simulink model "HumanPilot"  (R2023b)
settings: Solver=FixedStepAuto  StartTime=0.0  StopTime=inf  FixedStep=sample_time  RelTol=1e-3
model workspace (MAT data in the model file):
  SL_ROS_VariableLengthArrays_MaxSizes.CommonInfo.ArrayTruncateAction = 'EmitWarning'
  SL_ROS_VariableLengthArrays_MaxSizes.MsgTypeMap = containers.Map
  SL_ROS_VariableLengthArrays_MaxSizes.MsgTypeMap.serialization.keys = {'sensor_msgs/Image'}
  SL_ROS_VariableLengthArrays_MaxSizes.MsgTypeMap.serialization.values{1}(1).PropertyName = 'data'
  SL_ROS_VariableLengthArrays_MaxSizes.MsgTypeMap.serialization.values{1}(1).DataType = 'uint8'
  SL_ROS_VariableLengthArrays_MaxSizes.MsgTypeMap.serialization.values{1}(1).MaxLength = 921600
  SL_ROS_VariableLengthArrays_MaxSizes.MsgTypeMap.serialization.values{1}(2).PropertyName = 'encoding'
  SL_ROS_VariableLengthArrays_MaxSizes.MsgTypeMap.serialization.values{1}(2).DataType = 'uint8'
  SL_ROS_VariableLengthArrays_MaxSizes.MsgTypeMap.serialization.values{1}(2).MaxLength = 128
  SL_ROS_VariableLengthArrays_MaxSizes.MsgTypeMap.serialization.uniformity = 0
  SL_ROS_VariableLengthArrays_MaxSizes.MsgTypeMap.serialization.keyType = 'char'
  SL_ROS_VariableLengthArrays_MaxSizes.MsgTypeMap.serialization.valueType = 'any'
  sample_time = 0.1
undefined symbols (not defined in the file): duration, vel
libraries: ros2lib x6, visionsinks x2, vrlib x1, simulink_extras x1
settings Model: Creator=rcasado  LastModifiedBy=Rafa
settings SolverCC: AlgebraicLoopSolver=TrustRegion
settings DataIOCC: ReturnWorkspaceOutputs=off
settings OptimizationCC: EnhancedBackFolding=on  PassReuseOutputArgsAs=Individual arguments  ZeroExternalMemoryAtStartup=off  ZeroInternalMemoryAtStartup=off  MaxStackSize=64  OptimizeBlockOrder=speed  DifferentSizesBufferReuse=on  OptimizationCustomize=off  EfficientTunableParamExpr=on
settings DebuggingCC: ParameterTunabilityLossMsg=error  UnconnectedInputMsg=warning  UnconnectedOutputMsg=warning  UnconnectedLineMsg=warning  BusObjectLabelMismatch=none  PregeneratedLibrarySubsystemCodeDiagnostic=none  ArithmeticOperatorsInVariantConditions=warning
settings HardwareCC: ProdBitPerPointer=32  ProdBitPerSizeT=32  ProdBitPerPtrDiffT=32  ProdLargestAtomicFloat=None  ProdIntDivRoundTo=Undefined  ProdEndianess=Unspecified  ProdWordSize=32  ProdHWDeviceType=Generic->Unspecified (assume 32-bit Generic)
settings ModelReferenceCC: EnableRefExpFcnMdlSchedulingChecks=on
settings SFSimCC: SimUseLocalCustomCode=off  CustomCodeUndefinedFunction=UseInterfaceOnly  SimTargetLang=C++
settings RTWCC: Description=Embedded Coder  SystemTargetFile=ert.tlc  HardwareBoard=Robot Operating System (ROS)  TLCOptions="-aInlineSetEventsForThisBaseRateFcn=TLC_FALSE -aSuppressMultiTaskScheduler=TLC_FALSE  -aRateBasedStepFcn=0"  TemplateMakefile=ert_default_tmf  GenerateReport=on  RTWUseLocalCustomCode=off  Toolchain=Catkin  IncludeHyperlinkInReport=on  LaunchReport=on  TargetLang=C++  GenerateTraceInfo=on  GenerateTraceReport=on  GenerateTraceReportSl=on  GenerateTraceReportSf=on  GenerateTraceReportEml=on  DLArmComputeVersion=19.05
settings CodeAppCC: ForceParamTrailComments=on  IgnoreCustomStorageClasses=off  OperatorAnnotations=on  SimulinkDataObjDesc=on  SFDataObjDesc=on  InsertBlockDesc=on

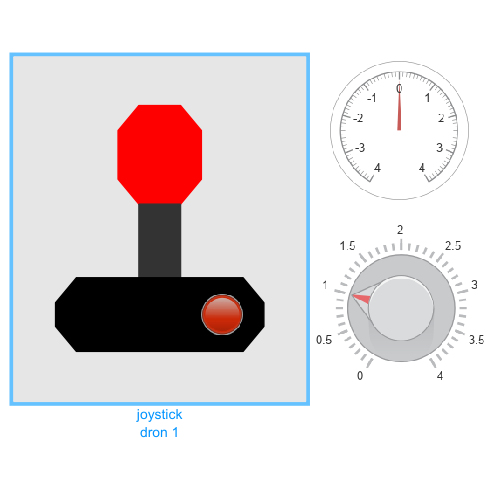
[thumbnail: Simulink's stored preview of the top-level diagram]
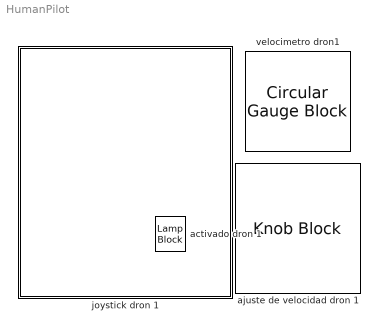
== system HumanPilot ==
  activado dron 1 : LampBlock  LabelPosition=Hide
  ajuste de velocidad dron 1 : KnobBlock  LabelPosition=Hide  ScaleMax=4  TickInterval=0.5
  joystick dron 1 : Subsystem
      mask Display:
      | patch([12 -2 -2 12], [12 12 -2 -2], [0.9 0.9 0.9])
      | 
      | % bola roja
      | patch([4 6 7 7 6 4 3 3], [6 6 7 9 10 10 9 7], [1 0 0])
      | 
      | % palo gris
      | patch([4 6 6 4], [3 3 6 6], [0.2 0.2 0.2])
      | 
      | % base negra
      | patch([1 9 10 10 9 1 0 0], [0 0 1 2 3 3 2 1], [0 0 0])
  velocimetro dron1 : CircularGaugeBlock  LabelPosition=Hide  ScaleMin=-4  ScaleMax=4  TickInterval=1

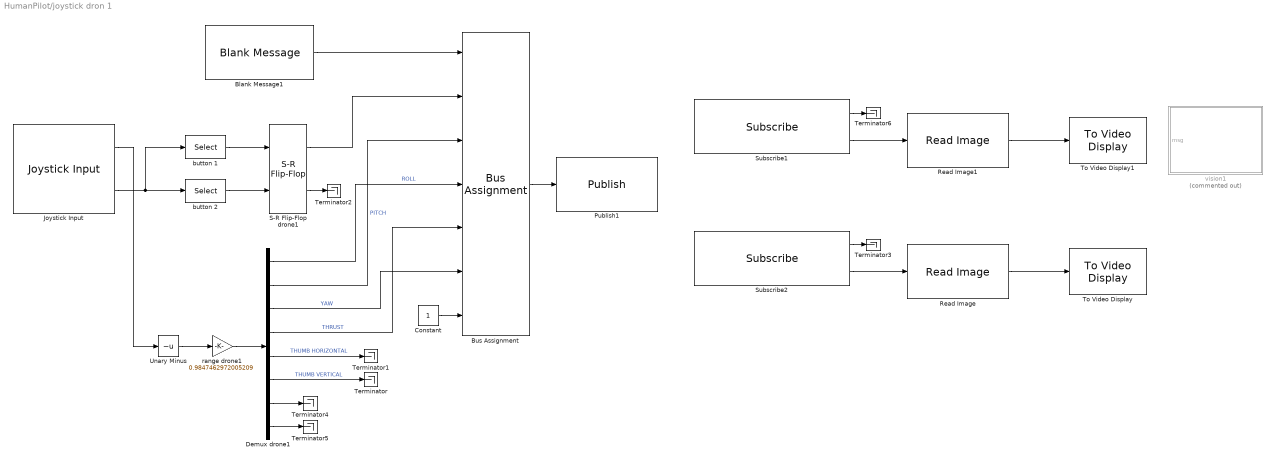
== system HumanPilot/joystick dron 1 ==
  Blank Message1 : ros2lib/Blank Message  messageClass=Message  entityType=navsim_msgs/RemoteCommand  messageType=navsim_msgs/RemoteCommand  SampleTime=sample_time
  Bus Assignment : BusAssignment  AssignedSignals=on,vel.linear.x,vel.linear.y,vel.linear.z,vel.angular.z,duration.sec
  Constant : Constant  OutDataTypeStr=int32
  Demux drone1 : Demux  Outputs=8
  Joystick Input : vrlib/Joystick Input  joyid=1  adjustports=off  forcefeed=off
  Publish1 : ros2lib/Publish  topicSource=Select from ROS network  topic=/UAV/abejorro1/RemoteCommand  messageType=navsim_msgs/RemoteCommand  QOSHistory=Keep last  QOSDepth=1  QOSReliability=Reliable  QOSDurability=Volatile
  Read Image : ros2lib/Read Image  MaximumImageSize=[320, 480]  ImageEncoding=rgb8  ShowAlphaOutput=off  ShowErrorCodeOutput=off  VariableSizeOutputs=off
  Read Image1 : ros2lib/Read Image  MaximumImageSize=[240, 320]  ImageEncoding=rgb8  ShowAlphaOutput=off  ShowErrorCodeOutput=off  VariableSizeOutputs=off
  S-R Flip-Flop drone1 : simulink_extras/Flip Flops/S-R Flip-Flop  initial_condition=0
  Subscribe1 : ros2lib/Subscribe  topicSource=Select from ROS network  topic=/UAV/abejorro1/onboard_cam/image_raw  messageType=sensor_msgs/Image  sampleTime=0.1  QOSHistory=Keep last  QOSDepth=1  QOSReliability=Reliable  QOSDurability=Volatile
  Subscribe2 : ros2lib/Subscribe  topicSource=Select from ROS network  topic=/UAV/abejorro1/follow_cam/image_raw  messageType=sensor_msgs/Image  sampleTime=0.1  QOSHistory=Keep last  QOSDepth=1  QOSReliability=Reliable  QOSDurability=Volatile
  Terminator{,1..6} (7 alike) : Terminator
  To Video Display : visionsinks/To Video Display  windowSizeMode=True size (1:1)  openAtMdlStart=on  fullScreen=off  videoWindowX=4122  videoWindowY=1148  saveWindowSize=off  videoWindowWidth=480  videoWindowHeight=320  inputColorFormat=RGB  inputType=Obsolete  imagePorts=One multidimensional signal  OutputDevice=On-screen video monitor  dataOrg=Column-major  isWindowOpen=off
  To Video Display1 : visionsinks/To Video Display  windowSizeMode=Normal  openAtMdlStart=on  fullScreen=off  videoWindowX=3600  videoWindowY=1154  saveWindowSize=off  videoWindowWidth=430  videoWindowHeight=322  inputColorFormat=RGB  inputType=Obsolete  imagePorts=One multidimensional signal  OutputDevice=On-screen video monitor  dataOrg=Column-major  isWindowOpen=off
  Unary Minus : UnaryMinus
  button 1 : Selector  InputPortWidth=32  IndexOptions=Index vector (dialog)  Indices=[1]  OutputSizes=1
  button 2 : Selector  InputPortWidth=32  IndexOptions=Index vector (dialog)  Indices=[2]  OutputSizes=1
  range drone1 : Gain  Gain=0.9847462972005209
  vision1 : MATLAB Function  Commented=on  TreatAsAtomicUnit=on
  wires:
  Bus Assignment/1 -> Publish1/1
  Blank Message1/1 -> Bus Assignment/1
  Joystick Input/1 -> Unary Minus/1
  Demux drone1/1 -> Bus Assignment/4  "ROLL"
  Demux drone1/2 -> Bus Assignment/3  "PITCH"
  Demux drone1/3 -> Bus Assignment/6  "YAW"
  Demux drone1/4 -> Bus Assignment/5  "THRUST"
  Demux drone1/5 -> Terminator1/1  "THUMB HORIZONTAL"
  Demux drone1/6 -> Terminator/1  "THUMB VERTICAL"
  Demux drone1/7 -> Terminator4/1
  Demux drone1/8 -> Terminator5/1
  Joystick Input/2 -> button 2/1, button 1/1
  S-R Flip-Flop drone1/1 -> Bus Assignment/2
  button 2/1 -> S-R Flip-Flop drone1/2
  button 1/1 -> S-R Flip-Flop drone1/1
  S-R Flip-Flop drone1/2 -> Terminator2/1
  Unary Minus/1 -> range drone1/1
  range drone1/1 -> Demux drone1/1
  Subscribe1/2 -> Read Image1/1
  Read Image1/1 -> To Video Display1/1
  Subscribe1/1 -> Terminator6/1
  Subscribe2/1 -> Terminator3/1
  Subscribe2/2 -> Read Image/1
  Read Image/1 -> To Video Display/1
  Constant/1 -> Bus Assignment/7

== matlab function HumanPilot/joystick dron 1/vision1 ==
  data: msg input
function fcn(msg)

% leemos la imagen
img = uint8(zeros(msg.height,msg.width,3));
elem = 1;
for fil = 1:msg.height
    for col = 1:msg.width
        for rgb = 1:3
            img(fil,col,rgb) = msg.data(elem);
            elem = elem + 1;
        end
    end
end

figName = 'Drone camera';
figHandler = findobj('Type','figure','Name',figName)';
    
if isempty(figHandler) 
    % la figura no existe, hay que construirla
    figure( ...
        'Name',figName, ...
        'NumberTitle','off', ...
        'MenuBar', 'none', ...
        'Resize','on');

    % eje dentro de la figura
%     axesHandler = axes(      ...
%       'Parent', figHandler,  ...
%       'Units','normalized', ...
%       'Visible','on');
%     grid(axesHandler,'on');
%     hold(axesHandler,'on');
%     axis equal
%     axis([-160 160 -120 120])

end


coder.extrinsic('image');
image(img);
